simulink model "suspensao_traseira_pibit_2025"  (R2025a)
settings: Solver=VariableStepAuto  StartTime=0.0  StopTime=10.0  RelTol=1e-3
values from neighbouring files (symbols this model uses):
  bp = 5    [parametros_suspensao_completo_pibit.m]    (also in parametros_suspensao_completo_pibit_final.m)
  bs = 10    [parametros_suspensao_completo_pibit.m]    (also in parametros_suspensao_completo_pibit_final.m)
  g = 9.81    [parametros_suspensao_completo_pibit.m]    (also in parametros_suspensao_completo_pibit_final.m)
  I = 5.6e-4    (= 0.00056)    [parametros_suspensao_completo_pibit.m]    (also in parametros_suspensao_completo_pibit_final.m)
  kp = 1000    [parametros_suspensao_completo_pibit.m]    (also in parametros_suspensao_completo_pibit_final.m)
  ks = 200    [parametros_suspensao_completo_pibit.m]    (also in parametros_suspensao_completo_pibit_final.m)
  massa_nao_suspensa = 200/1000    (= 0.2)    [parametros_suspensao_completo_pibit.m]    (also in parametros_suspensao_completo_pibit_final.m)

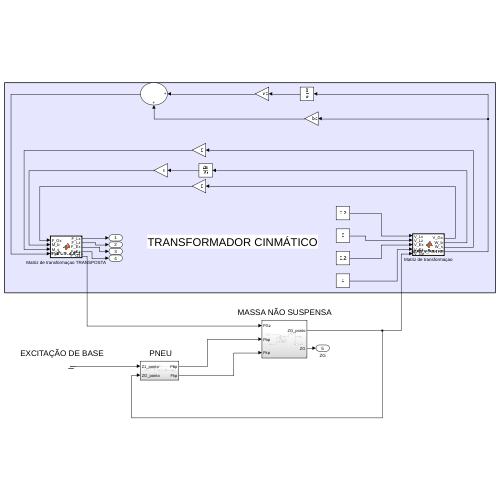
[thumbnail: Simulink's stored preview of the top-level diagram]
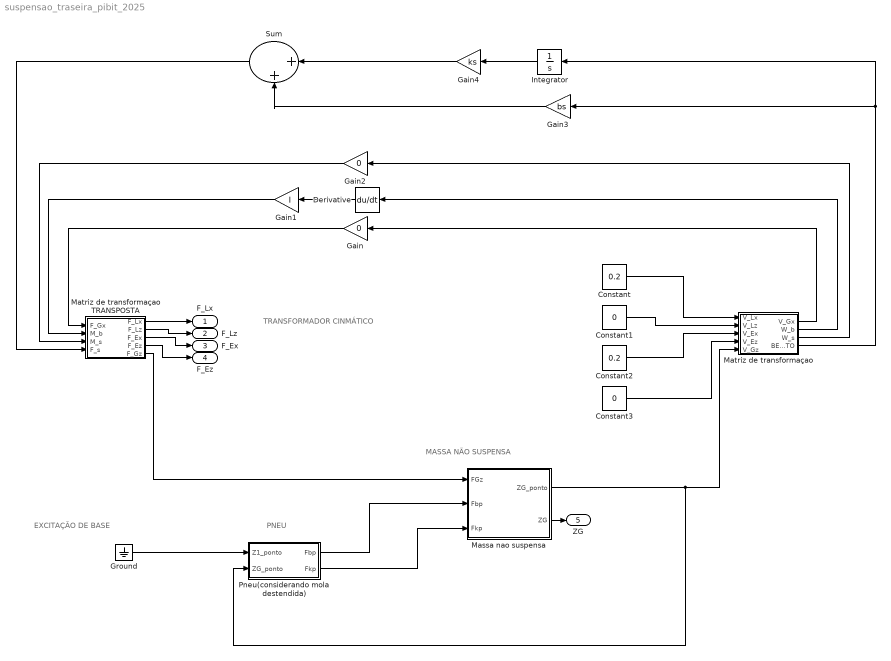
== system suspensao_traseira_pibit_2025 ==
  note: EXCITAÇÃO DE BASE
  note: MASSA NÃO SUSPENSA
  note: PNEU
  note: TRANSFORMADOR CINMÁTICO
  Constant : Constant  Value=0.2
  Constant1 : Constant  Value=0
  Constant2 : Constant  Value=0.2
  Constant3 : Constant  Value=0
  Derivative : Derivative
  Gain : Gain  Gain=0
  Gain1 : Gain  Gain=I
  Gain2 : Gain  Gain=0
  Gain3 : Gain  Gain=bs
  Gain4 : Gain  Gain=ks
  Ground : Ground
  Integrator : Integrator
  Massa nao suspensa : Subsystem
  Matriz de transformaçao : MATLAB Function  TreatAsAtomicUnit=on
  Matriz de transformaçao TRANSPOSTA : MATLAB Function  TreatAsAtomicUnit=on
  Pneu(considerando mola destendida) : Subsystem
  Sum : Sum  Inputs=|++
  F_Lx : Outport
  F_Lz : Outport  Port=2
  F_Ex : Outport  Port=3
  F_Ez : Outport  Port=4
  ZG : Outport  Port=5
  wires:
  Matriz de transformaçao/1(V_Gx) -> Gain/1
  Matriz de transformaçao/3(W_s) -> Gain2/1
  Constant1/1 -> Matriz de transformaçao/2(V_Lz)
  Constant/1 -> Matriz de transformaçao/1(V_Lx)
  Constant3/1 -> Matriz de transformaçao/4(V_Ez)
  Constant2/1 -> Matriz de transformaçao/3(V_Ex)
  Matriz de transformaçao/2(W_b) -> Derivative/1
  Gain/1 -> Matriz de transformaçao TRANSPOSTA/1(F_Gx)
  Derivative/1 -> Gain1/1
  Gain1/1 -> Matriz de transformaçao TRANSPOSTA/2(M_b)
  Gain2/1 -> Matriz de transformaçao TRANSPOSTA/3(M_s)
  Sum/1 -> Matriz de transformaçao TRANSPOSTA/4(F_s)
  Matriz de transformaçao/4(BETA_1_PONTO) -> Gain3/1, Integrator/1
  Gain3/1 -> Sum/2
  Integrator/1 -> Gain4/1
  Gain4/1 -> Sum/1
  Massa nao suspensa/1(ZG_ponto) -> Pneu(considerando mola destendida)/2(ZG_ponto), Matriz de transformaçao/5(V_Gz)
  Matriz de transformaçao TRANSPOSTA/1(F_Lx) -> F_Lx/1
  Matriz de transformaçao TRANSPOSTA/2(F_Lz) -> F_Lz/1
  Matriz de transformaçao TRANSPOSTA/3(F_Ex) -> F_Ex/1
  Matriz de transformaçao TRANSPOSTA/4(F_Ez) -> F_Ez/1
  Pneu(considerando mola destendida)/1(Fbp) -> Massa nao suspensa/2(Fbp)
  Pneu(considerando mola destendida)/2(Fkp) -> Massa nao suspensa/3(Fkp)
  Ground/1 -> Pneu(considerando mola destendida)/1(Z1_ponto)
  Matriz de transformaçao TRANSPOSTA/5(F_Gz) -> Massa nao suspensa/1(FGz)
  Massa nao suspensa/2(ZG) -> ZG/1

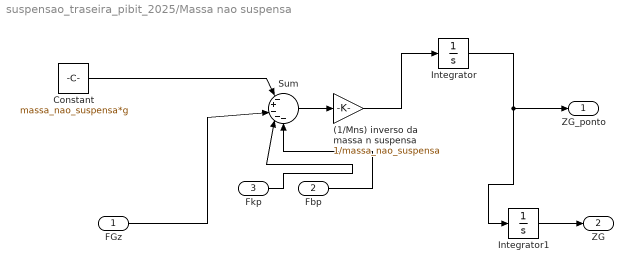
== system suspensao_traseira_pibit_2025/Massa nao suspensa ==
  FGz : Inport
  Fbp : Inport  Port=2
  Fkp : Inport  Port=3
  (1/Mns) inverso da massa n suspensa : Gain  Gain=1/massa_nao_suspensa
  Constant : Constant  Value=massa_nao_suspensa*g
  Integrator : Integrator
  Integrator1 : Integrator  InitialCondition=1
  Sum : Sum  Inputs=|-+---
  ZG_ponto : Outport
  ZG : Outport  Port=2
  wires:
  Integrator/1 -> Integrator1/1, ZG_ponto/1
  Fbp/1 -> Sum/5
  Fkp/1 -> Sum/4
  (1/Mns) inverso da massa n suspensa/1 -> Integrator/1
  Sum/1 -> (1/Mns) inverso da massa n suspensa/1
  FGz/1 -> Sum/3
  Constant/1 -> Sum/1
  Integrator1/1 -> ZG/1

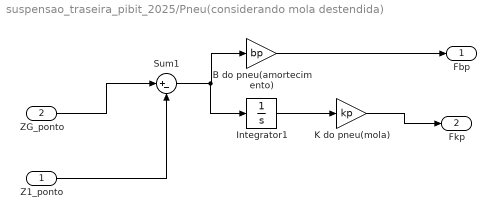
== system suspensao_traseira_pibit_2025/Pneu(considerando mola destendida) ==
  Z1_ponto : Inport
  ZG_ponto : Inport  Port=2
  B do pneu(amortecimento) : Gain  Gain=bp
  Integrator1 : Integrator
  K do pneu(mola) : Gain  Gain=kp
  Sum1 : Sum  Inputs=|+-
  Fbp : Outport
  Fkp : Outport  Port=2
  wires:
  Z1_ponto/1 -> Sum1/2
  ZG_ponto/1 -> Sum1/1
  Sum1/1 -> Integrator1/1, B do pneu(amortecimento)/1
  K do pneu(mola)/1 -> Fkp/1
  B do pneu(amortecimento)/1 -> Fbp/1
  Integrator1/1 -> K do pneu(mola)/1

== matlab function suspensao_traseira_pibit_2025/Matriz de transformaçao TRANSPOSTA ==
  data: F_Gx input; F_Lx output; M_b input; M_s input; F_s input; F_Lz output; F_Ex output; F_Ez output; F_Gz output
function [F_Lx, F_Lz, F_Ex, F_Ez, F_Gz] = minhaFuncaoForcas(F_Gx, M_b, M_s, F_s)
% Função para calcular as forças de saída usando a transposta da matriz M

    % Atribuir valores fixos para os parâmetros
    BETA_1 = 0.05465;    %fim de curso minimo 0.05465  % fim de curso maximo 0.0589 em metors
    BETA_2 = 2.729;  %fim de curso minimo 2.729 radianos %fim de curso maximo 2.591 radianos
    BETA_3 =  2.264; %fim de curso  2.264 radianos %fim de curso maximo 2.168 radianos
    GAMA = 0.3788; %metros
    R_1 = 0.091782; %metros
    R_2 = 0.048414; %metors

    % Defina a matriz de parâmetros da suspensão (mesma matriz M do código original)
    M = [
        0, 0, 1, -tan(BETA_2), tan(BETA_2);
        0, 0, 0, 1 / (R_1 * cos(BETA_2)), -1 / (R_1 * cos(BETA_2));
        sin(BETA_3) / BETA_1, cos(BETA_3) / BETA_1, -sin(BETA_3) / BETA_1, ...
        (R_2 * cos(BETA_2 + GAMA - BETA_3) / (R_1 * cos(BETA_2) * BETA_1)) - cos(BETA_3) / BETA_1, ...
        -R_2 * cos(BETA_2 + GAMA - BETA_3) / (R_1 * cos(BETA_2) * BETA_1);
        -cos(BETA_3), sin(BETA_3), cos(BETA_3), ...
        (R_2 * sin(-(BETA_2 + GAMA) + BETA_3) / (R_1 * cos(BETA_2))) - sin(BETA_3), ...
        R_2 * sin((BETA_2 + GAMA) - BETA_3) / (R_1 * cos(BETA_2))
    ];

    % Calcule a transposta da matriz M
    M_transposta = M';

    % Calcule os resultados multiplicando a matriz transposta pelos vetores de entrada
    resultado = M_transposta * [F_Gx; M_b; M_s; F_s];

    % Atribua os valores de saída
    F_Lx = resultado(1);
    F_Lz = resultado(2);
    F_Ex = resultado(3);
    F_Ez = resultado(4);
    F_Gz = resultado(5);
end

== matlab function suspensao_traseira_pibit_2025/Matriz de transformaçao ==
  data: V_Lx input; V_Gx output; V_Lz input; V_Ex input; V_Ez input; V_Gz input; W_b output; W_s output; BETA_1_PONTO output
function [V_Gx, W_b, W_s, BETA_1_PONTO] = minhaFuncao(V_Lx, V_Lz, V_Ex, V_Ez, V_Gz)
% Função para calcular variáveis de saída da suspensão a partir de múltiplas entradas

     % Atribuir valores fixos para os parâmetros
    BETA_1 = 0.05465;    %fim de curso minimo 0.05465  % fim de curso maximo 0.0589 em metors
    BETA_2 = 2.729;  %fim de curso minimo 2.729 radianos %fim de curso maximo 2.591 radianos
    BETA_3 =  2.264; %fim de curso  2.264 radianos %fim de curso maximo 2.168 radianos
    GAMA =  0.380; %radianos
    R_1 = 0.091782; %metros
    R_2 = 0.048414; %metors

    % Defina a matriz de parâmetros da suspensão
    M = [
        0, 0, 1, -tan(BETA_2), tan(BETA_2);
        0, 0, 0, 1 / (R_1 * cos(BETA_2)), -1 / (R_1 * cos(BETA_2));
        sin(BETA_3) / BETA_1, cos(BETA_3) / BETA_1, -sin(BETA_3) / BETA_1, ...
        (R_2 * cos(BETA_2 + GAMA - BETA_3) / (R_1 * cos(BETA_2) * BETA_1)) - cos(BETA_3) / BETA_1, ...
        -R_2 * cos(BETA_2 + GAMA - BETA_3) / (R_1 * cos(BETA_2) * BETA_1);
        -cos(BETA_3), sin(BETA_3), cos(BETA_3), ...
        (R_2 * sin(-(BETA_2 + GAMA) + BETA_3) / (R_1 * cos(BETA_2))) - sin(BETA_3), ...
        R_2 * sin((BETA_2 + GAMA) - BETA_3) / (R_1 * cos(BETA_2))
    ];

    % Calcule as saídas
    resultado = M * [V_Lx; V_Lz; V_Ex; V_Ez; V_Gz];

    % Atribua os valores de saída
    V_Gx = resultado(1);
    W_b = resultado(2);
    W_s = resultado(3); 
    BETA_1_PONTO = resultado(4); 
end
